simulink model "DelayLogic"  (R2023b)
settings: Solver=VariableStepAuto  StartTime=0.0  StopTime=10.0  RelTol=1e-3
undefined symbols (not defined in the file): SSR
libraries: dspswit3 x1
settings Model: Creator=sdegala  LastModifiedBy=sdegala

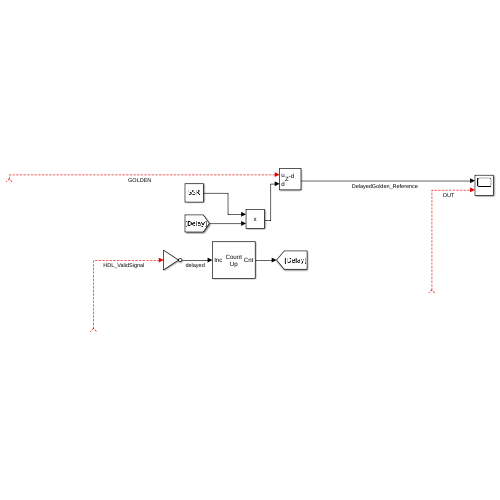
[thumbnail: Simulink's stored preview of the top-level diagram]
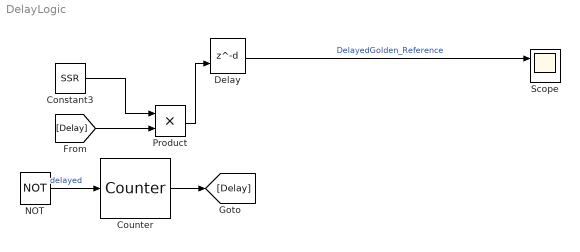
== system DelayLogic ==
  Constant3 : Constant  Value=SSR
  Counter : dspswit3/Counter  Direction=Up  CountEvent=Non-zero sample  CounterSize=User defined  MaxCount=10000  InitialCount=0  Output=Count  HitValue=32  ResetInput=off  SamplesPerFrame=1  Ts=1  CntDtype=double  HitDtype=Logical
  Delay : Delay  DelayLengthSource=Input port  DelayLengthUpperLimit=10000  InputProcessing=Columns as channels (frame based)
      settings: InputPortMap=u0,p1
  NOT : Logic  Operator=NOT  IconShape=distinctive  AllPortsSameDT=off  OutDataTypeStr=boolean
  Product : Product
  Scope : Scope  NumInputPorts=2
  wires:
  Delay/1 -> Scope/1  "DelayedGolden_Reference"
  Counter/1 -> [Delay]
  Product/1 -> Delay/2
  [Delay] -> Product/2
  Constant3/1 -> Product/1
  NOT/1 -> Counter/1  "delayed"
  ? -> Delay/1  "GOLDEN"
  ? -> NOT/1  "HDL_ValidSignal"
  ? -> Scope/2  "DUT"
